simulink model "MCU_LuenbergerObserver_dsPIC33AK128MC106"  (R2024a)
settings: Solver=FixedStepDiscrete  StartTime=0.0  StopTime=inf  FixedStep=50e-6  RelTol=1e-3  EnableMultiTasking=on
undefined symbols (not defined in the file or in its folder): A0, A4, ADC, B0, C10, C11, C6, C7, C8, control, D11, D12, DiscIntNeverNeededParam, inverter, Max, MaxPer, motor, ms, NumBits1, NumBits2, P1, P17, P20, P39, P40, P41, P43, P44, P60, P61, Pin, PosRange1, PosRange2, PWM1_Trg1, Resol, s, Slope1, Slope2, us
libraries: simulink x34, MCHP_Blockset x18
(part 3 of 5)

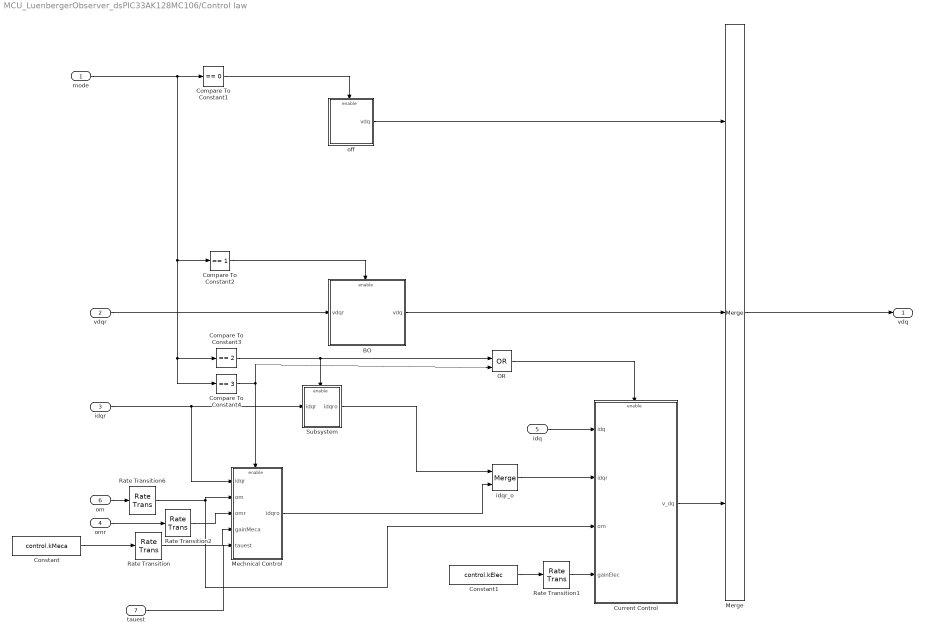
== system MCU_LuenbergerObserver_dsPIC33AK128MC106/Control law ==
  mode : Inport
  vdqr : Inport  Port=2
  idqr : Inport  Port=3
  omr : Inport  Port=4  PortDimensions=1
  idq : Inport  Port=5
  om : Inport  Port=6
  tauest : Inport  Port=7
  BO : Subsystem
  Compare To Constant1 : simulink/Logic and Bit Operations/Compare To Constant  relop===  const=0  OutDataTypeStr=boolean
  Compare To Constant2 : simulink/Logic and Bit Operations/Compare To Constant  relop===  const=1  OutDataTypeStr=boolean
  Compare To Constant3 : simulink/Logic and Bit Operations/Compare To Constant  relop===  const=2  OutDataTypeStr=boolean
  Compare To Constant4 : simulink/Logic and Bit Operations/Compare To Constant  relop===  const=3  OutDataTypeStr=boolean
  Constant : Constant  Value=control.kMeca  OutDataTypeStr=single
  Constant1 : Constant  Value=control.kElec  OutDataTypeStr=single
  Current Control : Subsystem  AncestorBlock=insa_control_base/Current Control
      settings: LibrarySourceBlock=insa_control_base/Current Control
  Mechnical Control : Subsystem
  Merge : Merge  Inputs=3
  OR : Logic  Operator=OR  IconShape=distinctive  AllPortsSameDT=off  OutDataTypeStr=boolean
  Rate Transition{,1..2,6} (4 alike) : RateTransition
  Subsystem : Subsystem
  idqr_o : Merge
  off : Subsystem
  vdq : Outport  VectorParamsAs1DForOutWhenUnconnected=off
  wires:
  Rate Transition6/1 -> Mechnical Control/2(om), Current Control/3(om)
  Rate Transition2/1 -> Mechnical Control/3(omr)
  Rate Transition1/1 -> Current Control/4(gainElec)
  Rate Transition/1 -> Mechnical Control/4(gainMeca)
  Constant1/1 -> Rate Transition1/1
  Constant/1 -> Rate Transition/1
  Merge/1 -> vdq/1
  BO/1(vdq) -> Merge/2
  Compare To Constant2/1 -> BO/Enable
  off/1(vdq) -> Merge/1
  Compare To Constant1/1 -> off/Enable
  Compare To Constant3/1 -> OR/1, Subsystem/Enable
  mode/1 -> Compare To Constant2/1, Compare To Constant3/1, Compare To Constant4/1, Compare To Constant1/1
  Subsystem/1(idqro) -> idqr_o/1
  Mechnical Control/1(idqro) -> idqr_o/2
  Compare To Constant4/1 -> OR/2, Mechnical Control/Enable
  om/1 -> Rate Transition6/1
  OR/1 -> Current Control/Enable
  idq/1 -> Current Control/1(idq)
  idqr_o/1 -> Current Control/2(idqr)
  Current Control/1(v_dq) -> Merge/3
  vdqr/1 -> BO/1(vdqr)
  idqr/1 -> Subsystem/1(idqr), Mechnical Control/1(idqr)
  omr/1 -> Rate Transition2/1
  tauest/1 -> Mechnical Control/5(tauest)

== system MCU_LuenbergerObserver_dsPIC33AK128MC106/Heart-beat 5Hz Blinking ==
  Delay : Delay  DelayLength=1  InitialCondition=0  SampleTime=.1
  Logical Operator : Logic  Operator=NOT  AllPortsSameDT=off  OutDataTypeStr=boolean
  Rate Transition2 : RateTransition  Deterministic=off  OutPortSampleTime=0.01
  LED1 : Outport  VectorParamsAs1DForOutWhenUnconnected=off
  wires:
  Rate Transition2/1 -> LED1/1
  Logical Operator/1 -> Rate Transition2/1, Delay/1
  Delay/1 -> Logical Operator/1

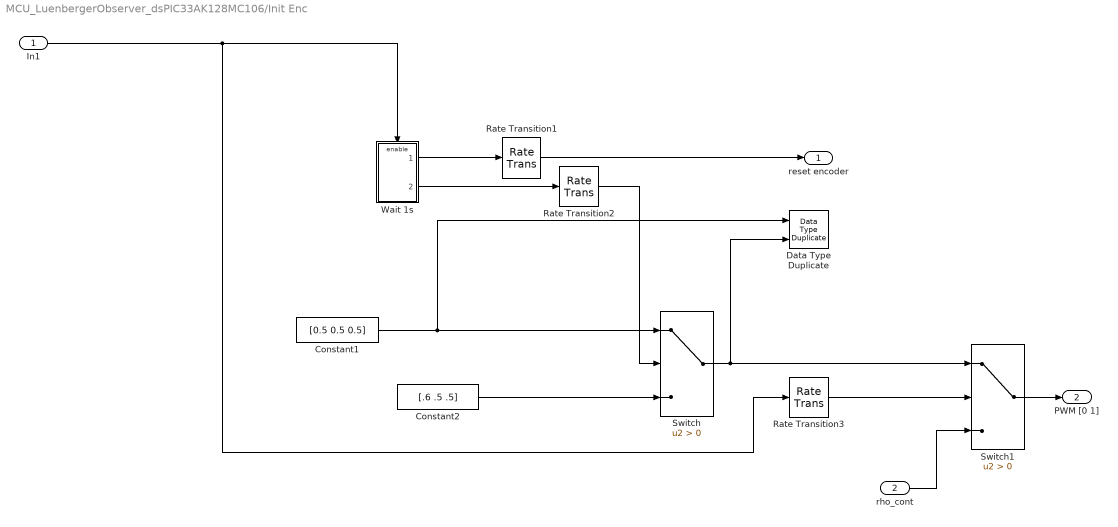
== system MCU_LuenbergerObserver_dsPIC33AK128MC106/Init Enc ==
  In1 : Inport
  rho_cont : Inport  Port=2
  Constant1 : Constant  Value=[0.5 0.5 0.5]  OutDataTypeStr=Inherit: Inherit via back propagation
  Constant2 : Constant  Value=[.6 .5 .5]  OutDataTypeStr=Inherit: Inherit via back propagation
  Data Type Duplicate : DataTypeDuplicate
  Rate Transition1 : RateTransition
  Rate Transition2 : RateTransition
  Rate Transition3 : RateTransition
  Switch : Switch  Criteria=u2 > Threshold  SaturateOnIntegerOverflow=off  InputSameDT=off
  Switch1 : Switch  Criteria=u2 > Threshold  SaturateOnIntegerOverflow=off  InputSameDT=off
  Wait 1s : Subsystem
  reset encoder : Outport
  PWM [0 1] : Outport  Port=2
  wires:
  Rate Transition3/1 -> Switch1/2
  In1/1 -> Rate Transition3/1, Wait 1s/Enable
  Wait 1s/1(init enc) -> Rate Transition1/1
  Constant1/1 -> Data Type Duplicate/1, Switch/1
  Switch/1 -> Switch1/1, Data Type Duplicate/2
  Wait 1s/2(init done) -> Rate Transition2/1
  Constant2/1 -> Switch/3
  rho_cont/1 -> Switch1/3
  Switch1/1 -> PWM [0 1]/1
  Rate Transition1/1 -> reset encoder/1
  Rate Transition2/1 -> Switch/2

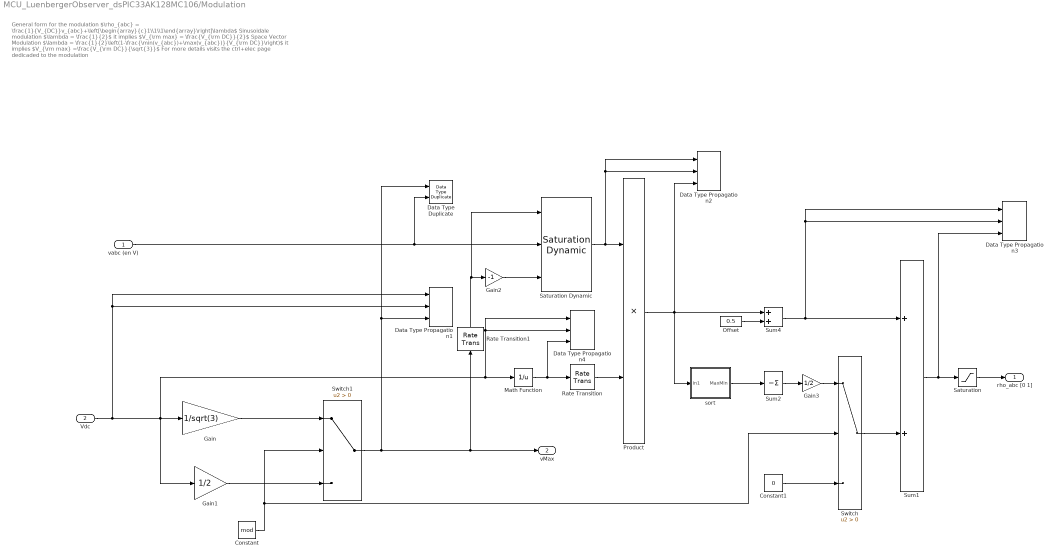
== system MCU_LuenbergerObserver_dsPIC33AK128MC106/Modulation ==
  note: General form for the modulation
      | $\rho_{abc} = \frac{1}{V_{DC}}v_{abc}+\left[\begin{array}{c}1\\1\\1\end{array}\right]\lambda$
      | Sinusoidale modulation
      | $\lambda = \frac{1}{2}$ it implies $V_{\rm max} = \frac{V_{\rm DC}}{2}$
      | Space Vector Modulation
      | $\lambda = \frac{1}{2}\left(1-\frac{\min(v_{abc})+\max(v_{abc})}{V_{\rm DC}}\right)$ it implies $V_{\rm max} =\frac{V_{\rm DC}}{\sqrt{3}}$
      | For more details visits the ctrl+elec page dedicaded to the modulation
  "vabc (en V) " : Inport
  Vdc : Inport  Port=2
  Constant : Constant  Value=mod  OutDataTypeStr=boolean
  Constant1 : Constant  Value=0  OutDataTypeStr=Inherit: Inherit via back propagation
  Data Type Duplicate : DataTypeDuplicate
  Data Type Propagation1 : simulink/Signal Attributes/Data Type Propagation  PropDataType=fixdt(1, 16)  IfRefDouble=double  IfRefSingle=single  IsSigned=TRUE  NumBitsBase=max([NumBits1 NumBits2])  NumBitsMult=1  NumBitsAdd=0  NumBitsAllowFinal=[1:128]  PropScaling=2^-(15-ceil(log2(inverter.vDC/sqrt(3))))  ValuesUsedBestPrec=[100 -100]  SlopeBase=max([PosRange1 PosRange2])  SlopeMult=1/sqrt(3)  SlopeAdd=0  BiasBase=Bias1  BiasMult=1  BiasAdd=0
  Data Type Propagation2 : simulink/Signal Attributes/Data Type Propagation  PropDataType=fixdt(1, 16)  IfRefDouble=double  IfRefSingle=single  IsSigned=TRUE  NumBitsBase=max([NumBits1 NumBits2])  NumBitsMult=1  NumBitsAdd=0  NumBitsAllowFinal=[1:128]  PropScalingMode=Specify via dialog  PropScaling=2^-14  ValuesUsedBestPrec=[100 -100]  SlopeBase=Slope1/Slope2  SlopeMult=1  SlopeAdd=0  BiasBase=Bias1  BiasMult=1  BiasAdd=0
  Data Type Propagation3 : simulink/Signal Attributes/Data Type Propagation  PropDataType=fixdt(1, 16)  IfRefDouble=double  IfRefSingle=single  IsSigned=FALSE  NumBitsBase=max([NumBits1 NumBits2])  NumBitsMult=1  NumBitsAdd=0  NumBitsAllowFinal=[1:128]  PropScalingMode=Specify via dialog  PropScaling=2^-14  ValuesUsedBestPrec=[100 -100]  SlopeBase=Slope1/Slope2  SlopeMult=1  SlopeAdd=0  BiasBase=Bias1  BiasMult=1  BiasAdd=0
  Data Type Propagation4 : simulink/Signal Attributes/Data Type Propagation  PropDataType=fixdt(1, 16)  IfRefDouble=double  IfRefSingle=single  IsSigned=FALSE  NumBitsBase=max([NumBits1 NumBits2])  NumBitsMult=1  NumBitsAdd=0  NumBitsAllowFinal=[1:128]  PropScalingMode=Specify via dialog  PropScaling=2^-16  ValuesUsedBestPrec=[100 -100]  SlopeBase=max([PosRange1 PosRange2])  SlopeMult=1/sqrt(3)  SlopeAdd=0  BiasBase=Bias1  BiasMult=1  BiasAdd=0
  Gain : Gain  Gain=1/sqrt(3)  OutDataTypeStr=Inherit: Same as input
  Gain1 : Gain  Gain=1/2  OutDataTypeStr=Inherit: Same as input
  Gain2 : Gain  Gain=-1  ParamDataTypeStr=int16  OutDataTypeStr=Inherit: Inherit via back propagation
  Gain3 : Gain  Gain=1/2  OutDataTypeStr=Inherit: Same as input
  Math Function : Math  Operator=reciprocal  OutputSignalType=real  OutDataTypeStr=Inherit: Inherit via back propagation  SaturateOnIntegerOverflow=off
  "Offset " : Constant  Value=0.5  OutMin=[0]  OutMax=[1]  OutDataTypeStr=Inherit: Inherit via back propagation
  Product : Product  Inputs=**  OutDataTypeStr=Inherit: Inherit via back propagation  SaturateOnIntegerOverflow=on
  Rate Transition : RateTransition
  Rate Transition1 : RateTransition
  Saturation : Saturate  UpperLimit=1  LowerLimit=0
  Saturation Dynamic : simulink/Discontinuities/Saturation Dynamic  OutMin=[]  OutMax=[]  OutDataTypeStr=Inherit: Same as second input  OutDataType=fixdt(1, 16)  OutScaling=2^-10  DoSatur=off
  Sum1 : Sum  OutMin=[0]  OutMax=[1]  OutDataTypeStr=Inherit: Inherit via back propagation  InputSameDT=on  SaturateOnIntegerOverflow=on
  Sum2 : Sum  Inputs=-  OutMin=[-1]  OutMax=[1]  InputSameDT=on  SaturateOnIntegerOverflow=on  OutDataTypeStr=Inherit: Same as first input
  Sum4 : Sum  OutMin=[-1]  OutMax=[1]  InputSameDT=on  SaturateOnIntegerOverflow=on  OutDataTypeStr=Inherit: Same as first input
  Switch : Switch  Criteria=u2 > Threshold  SaturateOnIntegerOverflow=off  InputSameDT=off
  Switch1 : Switch  Criteria=u2 > Threshold  OutDataTypeStr=Inherit: Inherit via back propagation  SaturateOnIntegerOverflow=off  InputSameDT=off
  sort : Subsystem
  rho_abc [0 1] : Outport  VectorParamsAs1DForOutWhenUnconnected=off
  vMax : Outport  Port=2  VectorParamsAs1DForOutWhenUnconnected=off
  wires:
  Rate Transition1/1 -> Gain2/1, Saturation Dynamic/1
  Rate Transition/1 -> Product/2
  "vabc (en V) "/1 -> Saturation Dynamic/2, Data Type Duplicate/2
  Constant/1 -> Switch/2, Switch1/2
  Switch1/1 -> Data Type Duplicate/1, Data Type Propagation1/3, vMax/1, Rate Transition1/1
  Math Function/1 -> Rate Transition/1, Data Type Propagation4/3
  Gain2/1 -> Saturation Dynamic/3
  Product/1 -> sort/1(In1), Sum4/1, Data Type Propagation2/3
  "Offset "/1 -> Sum4/2
  Switch/1 -> Sum1/2
  Constant1/1 -> Switch/3
  Sum4/1 -> Sum1/1, Data Type Propagation3/1, Data Type Propagation3/2
  Sum2/1 -> Gain3/1
  sort/1(MaxMin) -> Sum2/1
  Gain/1 -> Switch1/1
  Gain1/1 -> Switch1/3
  Saturation Dynamic/1 -> Data Type Propagation2/2, Data Type Propagation2/1, Product/1
  Saturation/1 -> rho_abc [0 1]/1
  Gain3/1 -> Switch/1
  Vdc/1 -> Gain1/1, Data Type Propagation4/1, Data Type Propagation4/2, Math Function/1, Gain/1, Data Type Propagation1/1, Data Type Propagation1/2
  Sum1/1 -> Data Type Propagation3/3, Saturation/1

== system MCU_LuenbergerObserver_dsPIC33AK128MC106/Park ==
  xab(c) : Inport
  P(pth) : Inport  Port=2
  Clarke : Subsystem
  Park : Subsystem
  idq : Outport
  wires:
  Park/1(xdq) -> idq/1  "idq"
  P(pth)/1 -> Park/2(P(pth))
  xab(c)/1 -> Clarke/1(xab(c))
  Clarke/1(xalphabeta) -> Park/1(xalphabeta)

== system MCU_LuenbergerObserver_dsPIC33AK128MC106/Park inverse ==
  xdq : Inport
  P(pth) : Inport  Port=2
  Clarke Inverse : Subsystem
  Park inverse : Subsystem
  xabc : Outport
  wires:
  Park inverse/1(xalpahbeta) -> Clarke Inverse/1(xalphabeta)
  xdq/1 -> Park inverse/1(xdq)
  Clarke Inverse/1(xabc) -> xabc/1
  P(pth)/1 -> Park inverse/2(P(pth))

== system MCU_LuenbergerObserver_dsPIC33AK128MC106/Rot ==
  sin cos : Inport
  Demux3 : Demux  Outputs=2
  Gain : Gain  Gain=-1  OutDataTypeStr=Inherit: Same as input
  Mux1 : Mux
  Reshape : Reshape  OutputDimensionality=Customize  OutputDimensions=[2,2]
  "cos sin -sin cos " : Outport  PortDimensions=[2 2]
  wires:
  Reshape/1 -> "cos sin -sin cos "/1
  sin cos/1 -> Demux3/1
  Gain/1 -> Mux1/2
  Mux1/1 -> Reshape/1
  Demux3/1 -> Mux1/3, Gain/1
  Demux3/2 -> Mux1/4, Mux1/1
